simulink library "adeye_lib"  (R2019a)
settings: Solver=VariableStepAuto  StartTime=0.0  StopTime=10.0  RelTol=1e-3
undefined symbols (not defined in the file): AngularVelocity, Clock_, Data, Data_SL_Info, DiscIntNeverNeededParam, Encoding, Encoding_SL_Info, Header, Height, LinearAcceleration, Orientation, Pose, Step, Twist, Width
libraries: robotlib x47, $bdroot x46, simulink_extras x12, dspsrcs4 x6, dspindex x6, robotcorelib x2, aerolibutil x2, PreScanSimulinkLibrary x1
(part 2 of 4)

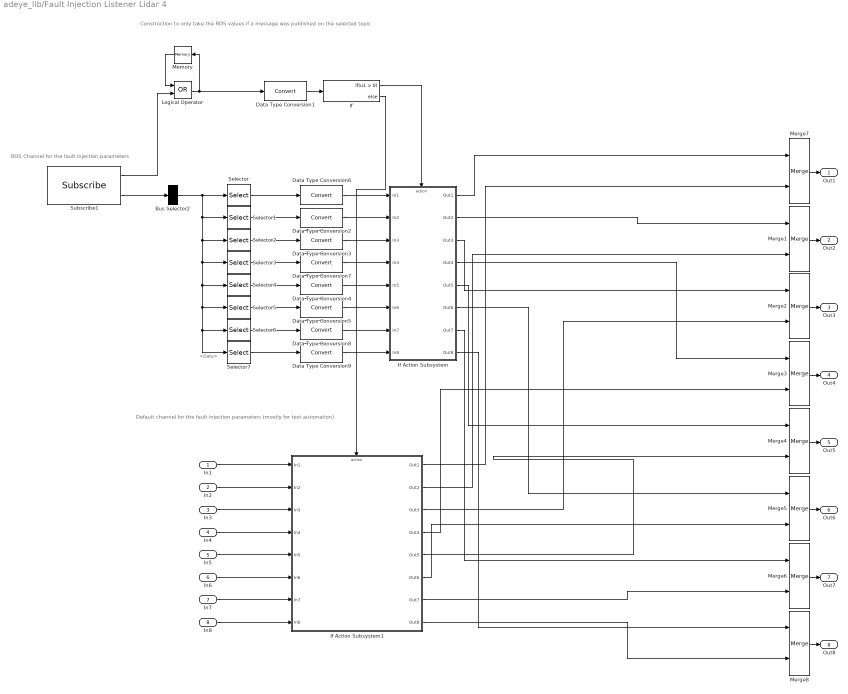
== system adeye_lib/Fault Injection Listener Lidar 4 ==
  note: Default channel for the fault injection parameters (mostly for test automation)
  note: ROS Channel for the fault injection parameters
  note: Construction to only take the ROS values if a message was published on the selected topic
  In1 : Inport
  In2 : Inport  Port=2
  In3 : Inport  Port=3
  In4 : Inport  Port=4
  In5 : Inport  Port=5
  In6 : Inport  Port=6
  In7 : Inport  Port=7
  In8 : Inport  Port=8
  Bus Selector2 : BusSelector  OutputSignals=Data
  Data Type Conversion{1..9} (9 alike) : DataTypeConversion
  If : If
  If Action Subsystem : Subsystem  TreatAsAtomicUnit=on
  If Action Subsystem1 : Subsystem  TreatAsAtomicUnit=on
  Logical Operator : Logic  Operator=OR  AllPortsSameDT=off  OutDataTypeStr=boolean
  Memory : Memory  InheritSampleTime=on
  Merge{1..8} (8 alike) : Merge
  Selector : Selector  InputPortWidth=128  IndexOptions=Index vector (dialog)  Indices=[1]  OutputSizes=1
  Selector1 : Selector  InputPortWidth=128  IndexOptions=Index vector (dialog)  Indices=[2]  OutputSizes=1
  Selector2 : Selector  InputPortWidth=128  IndexOptions=Index vector (dialog)  Indices=[3]  OutputSizes=1
  Selector3 : Selector  InputPortWidth=128  IndexOptions=Index vector (dialog)  Indices=[4]  OutputSizes=1
  Selector4 : Selector  InputPortWidth=128  IndexOptions=Index vector (dialog)  Indices=[5]  OutputSizes=1
  Selector5 : Selector  InputPortWidth=128  IndexOptions=Index vector (dialog)  Indices=[6]  OutputSizes=1
  Selector6 : Selector  InputPortWidth=128  IndexOptions=Index vector (dialog)  Indices=[7]  OutputSizes=1
  Selector7 : Selector  InputPortWidth=128  IndexOptions=Index vector (dialog)  Indices=[8]  OutputSizes=1
  Subscribe1 : robotlib/Subscribe  topicSource=Specify your own  topic=/fault_injection/lidar4  messageType=std_msgs/Float64MultiArray  sampleTime=-1  messageQueueLength=1
      settings: SourceProductBaseCode=RO
  Out1 : Outport
  Out2 : Outport  Port=2
  Out3 : Outport  Port=3
  Out4 : Outport  Port=4
  Out5 : Outport  Port=5
  Out6 : Outport  Port=6
  Out7 : Outport  Port=7
  Out8 : Outport  Port=8
  wires:
  Data Type Conversion6/1 -> If Action Subsystem/1(In1)
  If Action Subsystem/1(Out1) -> Merge7/1
  If/2 -> If Action Subsystem1/Action
  Logical Operator/1 -> Data Type Conversion1/1, Memory/1
  Subscribe1/1 -> Logical Operator/2
  Memory/1 -> Logical Operator/1
  If/1 -> If Action Subsystem/Action
  Data Type Conversion1/1 -> If/1
  If Action Subsystem1/1(Out1) -> Merge7/2
  Subscribe1/2 -> Bus Selector2/1
  In1/1 -> If Action Subsystem1/1(In1)
  Merge7/1 -> Out1/1
  Merge1/1 -> Out2/1
  Merge2/1 -> Out3/1
  Merge3/1 -> Out4/1
  Merge4/1 -> Out5/1
  Merge5/1 -> Out6/1
  Merge6/1 -> Out7/1
  Merge8/1 -> Out8/1
  If Action Subsystem/2(Out2) -> Merge1/1
  If Action Subsystem/3(Out3) -> Merge2/1
  If Action Subsystem/4(Out4) -> Merge3/1
  If Action Subsystem/5(Out5) -> Merge4/1
  If Action Subsystem/6(Out6) -> Merge5/1
  If Action Subsystem/7(Out7) -> Merge6/1
  If Action Subsystem/8(Out8) -> Merge8/1
  If Action Subsystem1/8(Out8) -> Merge8/2
  If Action Subsystem1/7(Out7) -> Merge6/2
  If Action Subsystem1/6(Out6) -> Merge5/2
  If Action Subsystem1/5(Out5) -> Merge4/2
  If Action Subsystem1/4(Out4) -> Merge3/2
  If Action Subsystem1/3(Out3) -> Merge2/2
  If Action Subsystem1/2(Out2) -> Merge1/2
  In2/1 -> If Action Subsystem1/2(In2)
  In5/1 -> If Action Subsystem1/5(In5)
  In4/1 -> If Action Subsystem1/4(In4)
  In3/1 -> If Action Subsystem1/3(In3)
  In6/1 -> If Action Subsystem1/6(In6)
  In8/1 -> If Action Subsystem1/8(In8)
  In7/1 -> If Action Subsystem1/7(In7)
  Data Type Conversion2/1 -> If Action Subsystem/2(In2)
  Selector1/1 -> Data Type Conversion2/1
  Data Type Conversion3/1 -> If Action Subsystem/3(In3)
  Selector2/1 -> Data Type Conversion3/1
  Data Type Conversion9/1 -> If Action Subsystem/8(In8)
  Data Type Conversion8/1 -> If Action Subsystem/7(In7)
  Data Type Conversion5/1 -> If Action Subsystem/6(In6)
  Data Type Conversion4/1 -> If Action Subsystem/5(In5)
  Data Type Conversion7/1 -> If Action Subsystem/4(In4)
  Selector3/1 -> Data Type Conversion7/1
  Selector4/1 -> Data Type Conversion4/1
  Selector5/1 -> Data Type Conversion5/1
  Selector6/1 -> Data Type Conversion8/1
  Selector7/1 -> Data Type Conversion9/1
  Selector/1 -> Data Type Conversion6/1
  Bus Selector2/1 -> Selector7/1, Selector6/1, Selector5/1, Selector4/1, Selector3/1, Selector2/1, Selector1/1, Selector/1  "<Data>"

== system adeye_lib/Fault Injection Listener Radar ==
  note: Default channel for the fault injection parameters (mostly for test automation)
  note: ROS Channel for the fault injection parameters
  note: Construction to only take the ROS values if a message was published on the selected topic
  State : Inport
  range_variance : Inport  Port=2
  theta_variance : Inport  Port=3
  phi_variance : Inport  Port=4
  Bus Selector2 : BusSelector  OutputSignals=Data
  Data Type Conversion{1..4,6} (5 alike) : DataTypeConversion
  If : If
  If Action Subsystem : Subsystem  TreatAsAtomicUnit=on
  If Action Subsystem1 : Subsystem  TreatAsAtomicUnit=on
  Logical Operator : Logic  Operator=OR  AllPortsSameDT=off  OutDataTypeStr=boolean
  Memory : Memory  InheritSampleTime=on
  Merge{1..3,7} (4 alike) : Merge
  Selector{,1..3} (4 alike) : Selector  InputPortWidth=128  IndexOptions=Index vector (dialog)  Indices=[1]  OutputSizes=1
  Subscribe1 : robotlib/Subscribe  topicSource=Specify your own  topic=/fault_injection/radar  messageType=std_msgs/Float64MultiArray  sampleTime=-1  messageQueueLength=1
      settings: SourceProductBaseCode=RO
  Out1 : Outport
  Out2 : Outport  Port=2
  Out3 : Outport  Port=3
  Out4 : Outport  Port=4
  wires:
  Merge7/1 -> Out1/1
  State/1 -> If Action Subsystem1/1(In1)
  Subscribe1/2 -> Bus Selector2/1
  If Action Subsystem1/1(Out1) -> Merge7/2
  Data Type Conversion1/1 -> If/1
  If/1 -> If Action Subsystem/Action
  Memory/1 -> Logical Operator/1
  Subscribe1/1 -> Logical Operator/2
  Logical Operator/1 -> Memory/1, Data Type Conversion1/1
  If/2 -> If Action Subsystem1/Action
  If Action Subsystem/1(Out1) -> Merge7/1
  Data Type Conversion6/1 -> If Action Subsystem/1(In1)
  Selector/1 -> Data Type Conversion6/1
  Bus Selector2/1 -> Selector3/1, Selector2/1, Selector1/1, Selector/1  "<Data>"
  Merge1/1 -> Out2/1
  Merge2/1 -> Out3/1
  Merge3/1 -> Out4/1
  If Action Subsystem/2(Out2) -> Merge1/1
  If Action Subsystem/3(Out3) -> Merge2/1
  If Action Subsystem/4(Out4) -> Merge3/1
  If Action Subsystem1/2(Out2) -> Merge1/2
  If Action Subsystem1/3(Out3) -> Merge2/2
  If Action Subsystem1/4(Out4) -> Merge3/2
  Selector1/1 -> Data Type Conversion2/1
  Selector2/1 -> Data Type Conversion3/1
  Data Type Conversion2/1 -> If Action Subsystem/2(In2)
  Data Type Conversion3/1 -> If Action Subsystem/3(In3)
  Selector3/1 -> Data Type Conversion4/1
  Data Type Conversion4/1 -> If Action Subsystem/4(In4)
  range_variance/1 -> If Action Subsystem1/2(In2)
  theta_variance/1 -> If Action Subsystem1/3(In3)
  phi_variance/1 -> If Action Subsystem1/4(In4)

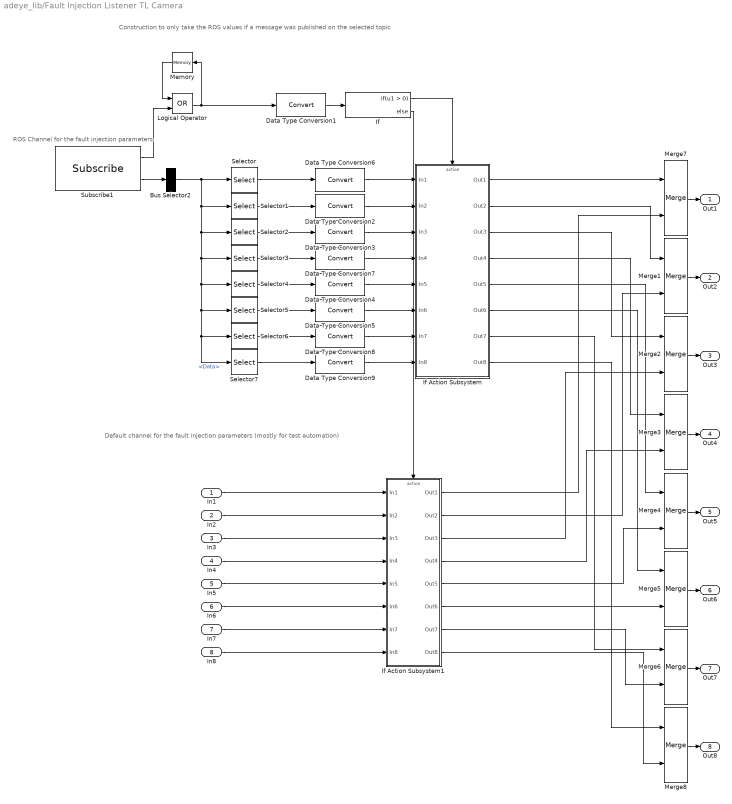
== system adeye_lib/Fault Injection Listener TL Camera ==
  note: Default channel for the fault injection parameters (mostly for test automation)
  note: ROS Channel for the fault injection parameters
  note: Construction to only take the ROS values if a message was published on the selected topic
  In1 : Inport
  In2 : Inport  Port=2
  In3 : Inport  Port=3
  In4 : Inport  Port=4
  In5 : Inport  Port=5
  In6 : Inport  Port=6
  In7 : Inport  Port=7
  In8 : Inport  Port=8
  Bus Selector2 : BusSelector  OutputSignals=Data
  Data Type Conversion{1..9} (9 alike) : DataTypeConversion
  If : If
  If Action Subsystem : Subsystem  TreatAsAtomicUnit=on
  If Action Subsystem1 : Subsystem  TreatAsAtomicUnit=on
  Logical Operator : Logic  Operator=OR  AllPortsSameDT=off  OutDataTypeStr=boolean
  Memory : Memory  InheritSampleTime=on
  Merge{1..8} (8 alike) : Merge
  Selector : Selector  InputPortWidth=128  IndexOptions=Index vector (dialog)  Indices=[1]  OutputSizes=1
  Selector1 : Selector  InputPortWidth=128  IndexOptions=Index vector (dialog)  Indices=[2]  OutputSizes=1
  Selector2 : Selector  InputPortWidth=128  IndexOptions=Index vector (dialog)  Indices=[3]  OutputSizes=1
  Selector3 : Selector  InputPortWidth=128  IndexOptions=Index vector (dialog)  Indices=[4]  OutputSizes=1
  Selector4 : Selector  InputPortWidth=128  IndexOptions=Index vector (dialog)  Indices=[5]  OutputSizes=1
  Selector5 : Selector  InputPortWidth=128  IndexOptions=Index vector (dialog)  Indices=[6]  OutputSizes=1
  Selector6 : Selector  InputPortWidth=128  IndexOptions=Index vector (dialog)  Indices=[7]  OutputSizes=1
  Selector7 : Selector  InputPortWidth=128  IndexOptions=Index vector (dialog)  Indices=[8]  OutputSizes=1
  Subscribe1 : robotlib/Subscribe  topicSource=Specify your own  topic=/fault_injection/tl_camera  messageType=std_msgs/Float64MultiArray  sampleTime=-1  messageQueueLength=1
      settings: SourceProductBaseCode=RO
  Out1 : Outport
  Out2 : Outport  Port=2
  Out3 : Outport  Port=3
  Out4 : Outport  Port=4
  Out5 : Outport  Port=5
  Out6 : Outport  Port=6
  Out7 : Outport  Port=7
  Out8 : Outport  Port=8
  wires:
  If Action Subsystem/1(Out1) -> Merge7/1
  If/2 -> If Action Subsystem1/Action
  Logical Operator/1 -> Data Type Conversion1/1, Memory/1
  Subscribe1/1 -> Logical Operator/2
  Memory/1 -> Logical Operator/1
  If/1 -> If Action Subsystem/Action
  Data Type Conversion1/1 -> If/1
  If Action Subsystem1/1(Out1) -> Merge7/2
  Subscribe1/2 -> Bus Selector2/1
  In1/1 -> If Action Subsystem1/1(In1)
  Merge7/1 -> Out1/1
  Selector/1 -> Data Type Conversion6/1
  Selector7/1 -> Data Type Conversion9/1
  Selector6/1 -> Data Type Conversion8/1
  Data Type Conversion4/1 -> If Action Subsystem/5(In5)
  Selector5/1 -> Data Type Conversion5/1
  Selector3/1 -> Data Type Conversion7/1
  Data Type Conversion5/1 -> If Action Subsystem/6(In6)
  Data Type Conversion7/1 -> If Action Subsystem/4(In4)
  Data Type Conversion8/1 -> If Action Subsystem/7(In7)
  Bus Selector2/1 -> Selector7/1, Selector6/1, Selector5/1, Selector4/1, Selector3/1, Selector2/1, Selector1/1, Selector/1  "<Data>"
  Data Type Conversion9/1 -> If Action Subsystem/8(In8)
  Selector4/1 -> Data Type Conversion4/1
  Selector1/1 -> Data Type Conversion2/1
  Data Type Conversion2/1 -> If Action Subsystem/2(In2)
  Data Type Conversion6/1 -> If Action Subsystem/1(In1)
  Selector2/1 -> Data Type Conversion3/1
  Data Type Conversion3/1 -> If Action Subsystem/3(In3)
  In2/1 -> If Action Subsystem1/2(In2)
  In3/1 -> If Action Subsystem1/3(In3)
  In4/1 -> If Action Subsystem1/4(In4)
  In5/1 -> If Action Subsystem1/5(In5)
  In6/1 -> If Action Subsystem1/6(In6)
  In7/1 -> If Action Subsystem1/7(In7)
  In8/1 -> If Action Subsystem1/8(In8)
  Merge1/1 -> Out2/1
  Merge2/1 -> Out3/1
  Merge3/1 -> Out4/1
  Merge4/1 -> Out5/1
  Merge5/1 -> Out6/1
  Merge6/1 -> Out7/1
  Merge8/1 -> Out8/1
  If Action Subsystem1/8(Out8) -> Merge8/2
  If Action Subsystem1/7(Out7) -> Merge6/2
  If Action Subsystem1/6(Out6) -> Merge5/2
  If Action Subsystem1/5(Out5) -> Merge4/2
  If Action Subsystem1/4(Out4) -> Merge3/2
  If Action Subsystem1/3(Out3) -> Merge2/2
  If Action Subsystem1/2(Out2) -> Merge1/2
  If Action Subsystem/2(Out2) -> Merge1/1
  If Action Subsystem/3(Out3) -> Merge2/1
  If Action Subsystem/8(Out8) -> Merge8/1
  If Action Subsystem/4(Out4) -> Merge3/1
  If Action Subsystem/5(Out5) -> Merge4/1
  If Action Subsystem/6(Out6) -> Merge5/1
  If Action Subsystem/7(Out7) -> Merge6/1

== system adeye_lib/Fault Injection Radar ==
  Range : Inport
  Theta : Inport  Port=2
  Phi : Inport  Port=3
  TargetTypeID : Inport  Port=4
  On/Off : Inport  Port=5
  range_variance : Inport  Port=6
  theta_variance : Inport  Port=7
  phi_variance : Inport  Port=8
  If : If
  If Action Subsystem : Subsystem  TreatAsAtomicUnit=on
  If Action Subsystem1 : Subsystem  TreatAsAtomicUnit=on
  Merge{,1..3} (4 alike) : Merge
  Out1 : Outport
  Out2 : Outport  Port=2
  Out3 : Outport  Port=3
  Out4 : Outport  Port=4
  wires:
  Merge/1 -> Out1/1
  Merge1/1 -> Out2/1
  Merge2/1 -> Out3/1
  If Action Subsystem/4(Out4) -> Merge3/1
  If Action Subsystem/3(Out3) -> Merge2/1
  If Action Subsystem/2(Out2) -> Merge1/1
  If Action Subsystem/1(Out1) -> Merge/1
  If Action Subsystem1/1(Out1) -> Merge/2
  If Action Subsystem1/2(Out2) -> Merge1/2
  If Action Subsystem1/3(Out3) -> Merge2/2
  If Action Subsystem1/4(Out4) -> Merge3/2
  Merge3/1 -> Out4/1
  On/Off/1 -> If/1
  TargetTypeID/1 -> If Action Subsystem1/4(In4), If Action Subsystem/4(In4)
  Phi/1 -> If Action Subsystem1/3(phi), If Action Subsystem/3(In3)
  Theta/1 -> If Action Subsystem/2(In2), If Action Subsystem1/2(theta)
  Range/1 -> If Action Subsystem1/1(range), If Action Subsystem/1(In1)
  If/1 -> If Action Subsystem1/Action
  If/2 -> If Action Subsystem/Action
  range_variance/1 -> If Action Subsystem1/5(range_variance)
  theta_variance/1 -> If Action Subsystem1/6(theta_variance)
  phi_variance/1 -> If Action Subsystem1/7(phi_variance)

== system adeye_lib/Lidar Adapter ==
  In1 : Inport
  In2 : Inport  Port=2
  In3 : Inport  Port=3
  In4 : Inport  Port=4
  In5 : Inport  Port=5
  Matrix Concatenate5 : Concatenate  NumInputs=4  Mode=Multidimensional array  ConcatenateDimension=2
  Reshape{1..4} (4 alike) : Reshape
  Rotate over Z : Subsystem
  Spherical to cartesian : Subsystem
  Out1 : Outport
  wires:
  In4/1 -> Reshape2/1
  In2/1 -> Reshape4/1
  Matrix Concatenate5/1 -> Out1/1
  Rotate over Z/1(Out1) -> Matrix Concatenate5/1
  Reshape3/1 -> Matrix Concatenate5/4
  Spherical to cartesian/3(Out3) -> Matrix Concatenate5/3
  Rotate over Z/2(Out2) -> Matrix Concatenate5/2
  In3/1 -> Reshape1/1
  Spherical to cartesian/2(Out2) -> Rotate over Z/3(In3)
  Reshape2/1 -> Spherical to cartesian/3(In3)
  Spherical to cartesian/1(Out1) -> Rotate over Z/2(In2)
  Reshape1/1 -> Spherical to cartesian/2(In2)
  In1/1 -> Rotate over Z/1(In1)
  Reshape4/1 -> Spherical to cartesian/1(In1)
  In5/1 -> Reshape3/1

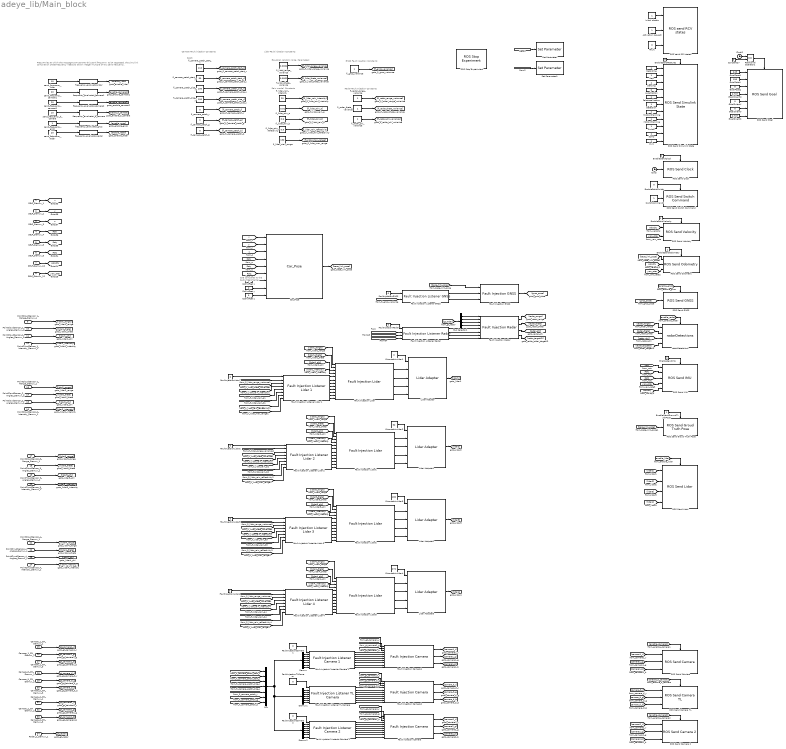
== system adeye_lib/Main_block ==
  note: Rain model, Constants
  note: Patch
  note: Lidar Fault injection Constants
  note: Camera Fault injection Constants
  note: Radar Fault Injection Constants
  note: Gaussian random noise, Parameters
  note: GNSS Fault Injection Constants
  note: CoG  compared
      | to the backwheels
      | center
  note: Frequencies at which the messages are sent
      |
      | For this send frequency to be respected, the simulink compilation sheet frequency
      | needs to be an integer multiple of this send frequency.
  SELF_Demux_1 : Inport
  SELF_Demux_2 : Inport  Port=2
  SELF_Demux_3 : Inport  Port=3
  SELF_Demux_4 : Inport  Port=4
  SELF_Demux_5 : Inport  Port=5
  SELF_Demux_6 : Inport  Port=6
  SELF_Demux_10 : Inport  Port=7
  SELF_Demux_12 : Inport  Port=8
  PointCloudSensor_1_Range_Demux_1 : Inport  Port=9
  PointCloudSensor_1_Angles_Demux_1 : Inport  Port=10
  PointCloudSensor_1_Angles_Demux_2 : Inport  Port=11
  PointCloudSensor_1_Intensity_Demux_1 : Inport  Port=12
  PointCloudSensor_2_Range_Demux_1 : Inport  Port=13
  PointCloudSensor_2_Angles_Demux_1 : Inport  Port=14
  PointCloudSensor_2_Angles_Demux_2 : Inport  Port=15
  PointCloudSensor_2_Intensity_Demux_1 : Inport  Port=16
  PointCloudSensor_3_Range_Demux_1 : Inport  Port=17
  PointCloudSensor_3_Angles_Demux_1 : Inport  Port=18
  PointCloudSensor_3_Angles_Demux_2 : Inport  Port=19
  PointCloudSensor_3_Intensity_Demux_1 : Inport  Port=20
  PointCloudSensor_4_Range_Demux_1 : Inport  Port=21
  PointCloudSensor_4_Angles_Demux_1 : Inport  Port=22
  PointCloudSensor_4_Angles_Demux_2 : Inport  Port=23
  PointCloudSensor_4_Intensity_Demux_1 : Inport  Port=24
  Camera_1_CM_Demux_1 : Inport  Port=25
  Camera_1_CM_Demux_2 : Inport  Port=26
  Camera_1_CM_Demux_3 : Inport  Port=27
  Camera_tl_CM_Demux_1 : Inport  Port=28
  Camera_tl_CM_Demux_2 : Inport  Port=29
  Camera_tl_CM_Demux_3 : Inport  Port=30
  Camera_2_CM_Demux_1 : Inport  Port=31
  Camera_2_CM_Demux_2 : Inport  Port=32
  Camera_2_CM_Demux_3 : Inport  Port=33
  Radar_1_Demux_1 : Inport  Port=34
  Activation request : Constant  OutDataTypeStr=Inherit: Inherit via back propagation
  Bus Selector1 : BusSelector  OutputSignals=Range[m],Theta[deg],Phi[deg],TargetTypeID[-]
  Car_Pose : $bdroot/Car_Pose  SystemSampleTime=-1
  Clock : Clock
  Clock2 : Clock
  CoG offset x : Constant  Value=0
  CoG offset y : Constant  Value=0
  CoG offset z : Constant  Value=0
  Constant27 : Constant  Value=0
  Demux : Demux  Outputs=7
  Demux1 : Demux  Outputs=7
  Demux2 : Demux  Outputs=7
  Detection : Constant
  EnableSendClock : Constant  OutDataTypeStr=Inherit: Inherit via back propagation
  EnableSendFeatures : Constant  Value=0  OutDataTypeStr=Inherit: Inherit via back propagation
  EnableSendGroundTruthPose : Constant
  EnableSendIMU : Constant  OutDataTypeStr=Inherit: Inherit via back propagation
  EnableSendOdometry : Constant
  EnableSendSwitch : Constant  Value=0  OutDataTypeStr=Inherit: Inherit via back propagation  SampleTime=0.05
  EnableSendVelocity : Constant  OutDataTypeStr=Inherit: Inherit via back propagation
  FakeLocalization : Constant
  Fault : Constant  Value=0  OutDataTypeStr=Inherit: Inherit via back propagation
  Fault Injection Camera : $bdroot/Fault Injection Camera  idy=200  idx=100  x=100  y=150  R=0  G=0  B=0
  Fault Injection Camera1 : $bdroot/Fault Injection Camera  idy=200  idx=100  x=100  y=150  R=0  G=0  B=0
  Fault Injection Camera2 : $bdroot/Fault Injection Camera  idy=200  idx=100  x=100  y=150  R=0  G=0  B=0
  Fault Injection GNSS : $bdroot/Fault Injection GNSS  f=20
  Fault Injection Lidar{,1..3} (4 alike) : $bdroot/Fault Injection Lidar  f=20  p=225*16
  Fault Injection Listener Camera 1 : $bdroot/Fault Injection Listener Camera 1  SystemSampleTime=-1
  Fault Injection Listener Camera 2 : $bdroot/Fault Injection Listener Camera 2  SystemSampleTime=-1
  Fault Injection Listener GNSS : $bdroot/Fault Injection Listener GNSS  SystemSampleTime=-1
  Fault Injection Listener Lidar 1 : $bdroot/Fault Injection Listener Lidar 1  SystemSampleTime=-1
  Fault Injection Listener Lidar 2 : $bdroot/Fault Injection Listener Lidar 2  SystemSampleTime=-1
  Fault Injection Listener Lidar 3 : $bdroot/Fault Injection Listener Lidar 3  SystemSampleTime=-1
  Fault Injection Listener Lidar 4 : $bdroot/Fault Injection Listener Lidar 4  SystemSampleTime=-1
  Fault Injection Listener Radar : $bdroot/Fault Injection Listener Radar  SystemSampleTime=-1
  Fault Injection Listener TL Camera : $bdroot/Fault Injection Listener TL Camera  SystemSampleTime=-1
  Fault Injection Radar : $bdroot/Fault Injection Radar  n=7
  FaultInjectionCamera1 : Constant  Value=0
  FaultInjectionCamera2 : Constant  Value=0
  FaultInjectionGNSS : Constant  Value=0  OutDataTypeStr=Inherit: Inherit via back propagation  SampleTime=0.05
  FaultInjectionLidar{1..4} (4 alike) : Constant  Value=0  OutDataTypeStr=Inherit: Inherit via back propagation
  FaultInjectionRadar : Constant  Value=0
  FaultInjectionTLCamera : Constant  Value=0
  GoalOrientW : Constant  Value=0.707
  GoalOrientX : Constant  Value=0
  GoalOrientY : Constant  Value=0
  GoalOrientZ : Constant  Value=0.707
  GoalPoseX : Constant  Value=249
  GoalPoseY : Constant  Value=136
  GoalPoseZ : Constant  Value=0
  Initial checks : Constant  OutDataTypeStr=Inherit: Inherit via back propagation
  Lidar Adapter{,1..3} (4 alike) : $bdroot/Lidar Adapter  SystemSampleTime=-1
  Localization : Constant  Value=0
  Map : Constant
  MissionPlanning : Constant
  MotionPlanning : Constant
  Mux : Mux  Inputs=7
  OrientationLidar1 : Constant  Value=0  OutDataTypeStr=Inherit: Inherit via back propagation
  OrientationLidar2 : Constant  Value=90  OutDataTypeStr=Inherit: Inherit via back propagation
  OrientationLidar3 : Constant  Value=180  OutDataTypeStr=Inherit: Inherit via back propagation
  OrientationLidar4 : Constant  Value=270  OutDataTypeStr=Inherit: Inherit via back propagation
  ROS Send Camera : $bdroot/ROS Send Camera  SystemSampleTime=-1
  ROS Send Camera 2 : $bdroot/ROS Send Camera 2  SystemSampleTime=-1
  ROS Send Camera TL : $bdroot/ROS Send Camera TL  SystemSampleTime=-1
  ROS Send Clock : $bdroot/ROS Send Clock  Priority=1  SystemSampleTime=-1
  ROS Send GNSS : $bdroot/ROS Send GNSS  SystemSampleTime=-1
  ROS Send Goal : $bdroot/ROS Send Goal  SystemSampleTime=-1
  ROS Send Groud Truth Pose : $bdroot/ROS Send Groud Truth Pose  SystemSampleTime=-1
  ROS Send IMU : $bdroot/ROS Send IMU  SystemSampleTime=-1
  ROS Send Lidar : $bdroot/ROS Send Lidar  SystemSampleTime=-1
  ROS Send Odometry : $bdroot/ROS Send Odometry  SystemSampleTime=-1
  ROS Send Simulink State : $bdroot/ROS Send Simulink State  SystemSampleTime=-1
  ROS Send Switch Command : $bdroot/ROS Send Switch Command  SystemSampleTime=-1
  ROS Send Velocity : $bdroot/ROS Send Velocity  SystemSampleTime=-1
  ROS Stop Experiment : $bdroot/ROS Stop Experiment  SystemSampleTime=-1
  ROS send RCV states : $bdroot/ROS send RCV states  SystemSampleTime=-1
  Recording : Constant
  Relational Operator1 : RelationalOperator  Operator===  OutDataTypeStr=boolean  RndMeth=Simplest
  Rviz : Constant
  Sensing : Constant
  Set Parameter : robotlib/Set Parameter  ParameterSource=Specify your own  ParameterName=/simulink/rain_intensity  ParameterType=double  ModelName=ROS_lib  BlockId=ParamSet_ROS_lib_3479
      settings: SourceProductName=Robotics System Toolbox  SourceProductBaseCode=RO
  Set Parameter1 : robotlib/Set Parameter  ParameterSource=Specify your own  ParameterName=/simulink/reflectivity  ParameterType=double  ModelName=ROS_lib  BlockId=ParamSet_ROS_lib_3480
      settings: SourceProductName=Robotics System Toolbox  SourceProductBaseCode=RO
  Ssmp : Constant
  Switch : Constant
  SwitchCommand : Constant  OutDataTypeStr=Inherit: Inherit via back propagation  SampleTime=0.05
  fi_camera_patch_b : Constant  Value=0
  fi_camera_patch_g : Constant  Value=0
  fi_camera_patch_r : Constant  Value=0
  fi_camera_patch_size_x : Constant  Value=100
  fi_camera_patch_size_y : Constant  Value=100
  fi_camera_patch_start_x : Constant  Value=110
  fi_camera_patch_start_y : Constant  Value=50
  fi_gnss_variance : Constant
  fi_lidar_max_range : Constant  Value=150
  fi_lidar_rain_a : Constant  Value=0.01
  fi_lidar_rain_b : Constant  Value=0.6
  fi_lidar_rain_intensity : Constant  Value=20
  fi_lidar_rain_reflectivity : Constant  Value=0.9
  fi_lidar_range_variance : Constant  Value=0.0001
  fi_lidar_theta_variance : Constant  Value=0.0001
  fi_radar_phi_variance : Constant
  fi_radar_range_variance : Constant
  fi_radar_theta_variance : Constant
  frequency_evaluator_camera1 : $bdroot/frequency_evaluator  SystemSampleTime=-1
  frequency_evaluator_camera2 : $bdroot/frequency_evaluator  SystemSampleTime=-1
  frequency_evaluator_gnss : $bdroot/frequency_evaluator  SystemSampleTime=-1
  frequency_evaluator_lidar : $bdroot/frequency_evaluator  SystemSampleTime=-1
      link override Constant: Value=0.999
  frequency_evaluator_radar : $bdroot/frequency_evaluator  SystemSampleTime=-1
  frequency_evaluator_tl_camera : $bdroot/frequency_evaluator  SystemSampleTime=-1
  radarDetections : $bdroot/radarDetections  SystemSampleTime=-1
  send_frequency_camera1 : Constant  Priority=1  Value=20
  send_frequency_camera2 : Constant  Priority=1  Value=20
  send_frequency_gnss : Constant  Priority=1
  send_frequency_lidar : Constant  Priority=1  Value=10
  send_frequency_radar : Constant  Priority=1  Value=20
  send_frequency_tl_camera : Constant  Priority=1  Value=10
  tag scope: Rotx=global, Roty=global, Rotz=global, velocity=global, x=global, y=global, yaw_rate=global, z=global
  wires:
  [p_refl_sfc] -> Set Parameter1/1
  [rain_intensity] -> Set Parameter/1
  Radar_1_Demux_1/1 -> [gt_radar]
  Camera_2_CM_Demux_3/1 -> [gt_camera2_b]
  Camera_2_CM_Demux_2/1 -> [gt_camera2_g]
  Camera_2_CM_Demux_1/1 -> [gt_camera2_r]
  SELF_Demux_10/1 -> [velocity]
  SELF_Demux_5/1 -> [Roty]
  SELF_Demux_12/1 -> [yaw_rate]
  SELF_Demux_4/1 -> [Rotx]
  SELF_Demux_1/1 -> [x]
  SELF_Demux_6/1 -> [Rotz]
  SELF_Demux_2/1 -> [y]
  SELF_Demux_3/1 -> [z]
  Camera_1_CM_Demux_1/1 -> [gt_camera1_r]
  Camera_1_CM_Demux_2/1 -> [gt_camera1_g]
  Camera_tl_CM_Demux_3/1 -> [gt_camera_tl_b]
  Camera_tl_CM_Demux_2/1 -> [gt_camera_tl_g]
  Camera_1_CM_Demux_3/1 -> [gt_camera1_b]
  Camera_tl_CM_Demux_1/1 -> [gt_camera_tl_r]
  GoalOrientW/1 -> ROS Send Goal/4
  GoalOrientX/1 -> ROS Send Goal/5
  GoalOrientY/1 -> ROS Send Goal/6
  Constant27/1 -> Relational Operator1/2
  Relational Operator1/1 -> ROS Send Goal/Enable
  Clock2/1 -> Relational Operator1/1
  GoalPoseZ/1 -> ROS Send Goal/3
  GoalPoseY/1 -> ROS Send Goal/2
  GoalOrientZ/1 -> ROS Send Goal/7
  GoalPoseX/1 -> ROS Send Goal/1
  EnableSendFeatures/1 -> ROS Send Simulink State/Enable
  [camera1_g] -> ROS Send Camera/2
  [camera1_b] -> ROS Send Camera/3
  [radar_phi] -> radarDetections/3
  [radar_range] -> radarDetections/1
  [velocity] -> ROS Send Odometry/2
  [gnss_pose] -> ROS Send GNSS/1
  MissionPlanning/1 -> ROS Send Simulink State/7
  [velocity] -> ROS Send Velocity/1
  EnableSendClock/1 -> ROS Send Clock/Enable
  Localization/1 -> ROS Send Simulink State/4
  Detection/1 -> ROS Send Simulink State/6
  FakeLocalization/1 -> ROS Send Simulink State/5
  [camera2_b] -> ROS Send Camera 2/3
  MotionPlanning/1 -> ROS Send Simulink State/8
  [camera1_r] -> ROS Send Camera/1
  [velocity] -> ROS Send IMU/5
  [camera_tl_b] -> ROS Send Camera TL/3
  [camera2_g] -> ROS Send Camera 2/2
  [camera2_r] -> ROS Send Camera 2/1
  [camera_tl_r] -> ROS Send Camera TL/1
  SwitchCommand/1 -> ROS Send Switch Command/1
  EnableSendVelocity/1 -> ROS Send Velocity/Enable
  Rviz/1 -> ROS Send Simulink State/11
  Switch/1 -> ROS Send Simulink State/9
  Recording/1 -> ROS Send Simulink State/1
  EnableSendOdometry/1 -> ROS Send Odometry/Enable
  Activation request/1 -> ROS send RCV states/2
  EnableSendSwitch/1 -> ROS Send Switch Command/Enable
  EnableSendIMU/1 -> ROS Send IMU/Enable
  [radar_targetID] -> radarDetections/4
  [yaw_rate] -> ROS Send IMU/4
  [lidar4] -> ROS Send Lidar/4
  Sensing/1 -> ROS Send Simulink State/3
  [yaw_rate] -> ROS Send Velocity/2
  [camera_tl_g] -> ROS Send Camera TL/2
  [Rotz] -> ROS Send IMU/3
  Fault/1 -> ROS send RCV states/3
  [Roty] -> ROS Send IMU/2
  Ssmp/1 -> ROS Send Simulink State/10
  [Rotx] -> ROS Send IMU/1
  [lidar2] -> ROS Send Lidar/2
  [radar_theta] -> radarDetections/2
  [yaw_rate] -> ROS Send Odometry/3
  [lidar3] -> ROS Send Lidar/3
  Clock/1 -> ROS Send Clock/1
  Map/1 -> ROS Send Simulink State/2
  Initial checks/1 -> ROS send RCV states/1
  [lidar1] -> ROS Send Lidar/1
  [base_link_pose] -> ROS Send Odometry/1
  fi_camera_patch_start_x/1 -> [fi_camera_patch_start_x]
  fi_camera_patch_start_y/1 -> [fi_camera_patch_start_y]
  fi_camera_patch_size_x/1 -> [fi_camera_patch_size_x]
  fi_radar_range_variance/1 -> [fi_radar_range_variance]
  fi_radar_theta_variance/1 -> [fi_radar_theta_variance]
  fi_lidar_range_variance/1 -> [fi_lidar_range_variance]
  fi_lidar_theta_variance/1 -> [fi_lidar_theta_variance]
  fi_radar_phi_variance/1 -> [fi_radar_phi_variance]
  fi_gnss_variance/1 -> [fi_gnss_variance]
  fi_camera_patch_g/1 -> [fi_camera_patch_g]
  fi_camera_patch_b/1 -> [fi_camera_patch_b]
  fi_lidar_rain_reflectivity/1 -> [fi_lidar_rain_reflectivity]
  fi_lidar_max_range/1 -> [fi_lidar_max_range]
  fi_camera_patch_r/1 -> [fi_camera_patch_r]
  fi_lidar_rain_a/1 -> [fi_lidar_rain_a]
  fi_lidar_rain_intensity/1 -> [fi_lidar_rain_intensity]
  fi_camera_patch_size_y/1 -> [fi_camera_patch_size_y]
  fi_lidar_rain_b/1 -> [fi_lidar_rain_b]
  PointCloudSensor_1_Range_Demux_1/1 -> [lidar1_range]
  PointCloudSensor_1_Angles_Demux_1/1 -> [lidar1_theta]
  PointCloudSensor_1_Angles_Demux_2/1 -> [lidar1_phi]
  PointCloudSensor_1_Intensity_Demux_1/1 -> [lidar1_intensity]
  PointCloudSensor_2_Range_Demux_1/1 -> [lidar2_range]
  PointCloudSensor_2_Angles_Demux_1/1 -> [lidar2_theta]
  PointCloudSensor_3_Range_Demux_1/1 -> [lidar3_range]
  PointCloudSensor_3_Angles_Demux_1/1 -> [lidar3_theta]
  PointCloudSensor_3_Angles_Demux_2/1 -> [lidar3_phi]
  PointCloudSensor_3_Intensity_Demux_1/1 -> [lidar3_intensity]
  PointCloudSensor_4_Range_Demux_1/1 -> [lidar4_range]
  PointCloudSensor_4_Angles_Demux_1/1 -> [lidar4_theta]
  PointCloudSensor_4_Intensity_Demux_1/1 -> [lidar4_intensity]
  PointCloudSensor_4_Angles_Demux_2/1 -> [lidar4_phi]
  PointCloudSensor_2_Angles_Demux_2/1 -> [lidar2_phi]
  PointCloudSensor_2_Intensity_Demux_1/1 -> [lidar2_intensity]
  OrientationLidar2/1 -> Lidar Adapter1/1
  Fault Injection Listener Radar/3 -> Fault Injection Radar/7
  Fault Injection Lidar3/4 -> Lidar Adapter3/5
  [fi_lidar_range_variance] -> Fault Injection Listener Lidar 3/2
  FaultInjectionLidar4/1 -> Fault Injection Listener Lidar 4/1
  [fi_lidar_rain_a] -> Fault Injection Listener Lidar 3/5
  [fi_lidar_theta_variance] -> Fault Injection Listener Lidar 4/3
  Fault Injection Camera/2 -> [camera2_g]
  Fault Injection Listener Lidar 4/2 -> Fault Injection Lidar3/6
  Fault Injection Camera2/3 -> [camera_tl_b]
  Fault Injection Camera1/1 -> [camera1_r]
  Fault Injection Camera/3 -> [camera2_b]
  [fi_lidar_rain_intensity] -> Fault Injection Listener Lidar 4/4
  [fi_lidar_rain_b] -> Fault Injection Listener Lidar 2/6
  Bus Selector1/4 -> Fault Injection Radar/4  "<TargetTypeID[-]>"
  [fi_lidar_rain_a] -> Fault Injection Listener Lidar 2/5
  Fault Injection Camera2/1 -> [camera_tl_r]
  [fi_lidar_rain_intensity] -> Fault Injection Listener Lidar 1/4
  Fault Injection Camera1/3 -> [camera1_b]
  Fault Injection Listener Lidar 3/6 -> Fault Injection Lidar2/10
  [lidar1_theta] -> Fault Injection Lidar/2
  [fi_lidar_max_range] -> Fault Injection Listener Lidar 1/8
  Fault Injection Camera2/2 -> [camera_tl_g]
  [lidar4_theta] -> Fault Injection Lidar3/2
  Fault Injection Listener Camera 2/3 -> Fault Injection Camera/6
  Fault Injection Lidar2/2 -> Lidar Adapter2/3
  Fault Injection Listener TL Camera/5 -> Fault Injection Camera2/8
  Fault Injection Radar/4 -> [radar_targetID]
  Fault Injection Radar/2 -> [radar_theta]
  [lidar1_phi] -> Fault Injection Lidar/3
  Fault Injection Listener Lidar 4/5 -> Fault Injection Lidar3/9
  [Roty] -> Car_Pose/5
  Fault Injection Listener Lidar 1/3 -> Fault Injection Lidar/7
  Fault Injection Listener Lidar 2/3 -> Fault Injection Lidar1/7
  [lidar2_theta] -> Fault Injection Lidar1/2
  [lidar4_phi] -> Fault Injection Lidar3/3
  Fault Injection Listener TL Camera/3 -> Fault Injection Camera2/6
  Fault Injection Listener Lidar 3/2 -> Fault Injection Lidar2/6
  Fault Injection Listener Camera 1/8 -> Fault Injection Camera1/11
  [lidar3_theta] -> Fault Injection Lidar2/2
  [lidar3_intensity] -> Fault Injection Lidar2/4
  Fault Injection Listener Lidar 3/1 -> Fault Injection Lidar2/5
  Bus Selector1/2 -> Fault Injection Radar/2  "<Theta[deg]>"
  Fault Injection Listener Lidar 2/7 -> Fault Injection Lidar1/11
  [gt_camera_tl_g] -> Fault Injection Camera2/2
  [lidar1_range] -> Fault Injection Lidar/1
  Fault Injection Lidar1/3 -> Lidar Adapter1/4
  [fi_lidar_rain_reflectivity] -> Fault Injection Listener Lidar 3/7
  [gt_camera_tl_r] -> Fault Injection Camera2/1
  [lidar3_range] -> Fault Injection Lidar2/1
  Fault Injection Listener Camera 1/6 -> Fault Injection Camera1/9
  Fault Injection Lidar2/3 -> Lidar Adapter2/4
  Lidar Adapter3/1 -> [lidar4]
  Fault Injection Listener Lidar 4/4 -> Fault Injection Lidar3/8
  [gt_camera_tl_b] -> Fault Injection Camera2/3
  Fault Injection Listener GNSS/2 -> Fault Injection GNSS/3
  Fault Injection Listener Lidar 2/8 -> Fault Injection Lidar1/12
  Fault Injection Lidar/3 -> Lidar Adapter/4
  Fault Injection Listener Radar/4 -> Fault Injection Radar/8
  [fi_radar_theta_variance] -> Fault Injection Listener Radar/3
  OrientationLidar4/1 -> Lidar Adapter3/1
  [fi_lidar_theta_variance] -> Fault Injection Listener Lidar 1/3
  Fault Injection Listener Camera 1/3 -> Fault Injection Camera1/6
  Fault Injection Listener Camera 1/4 -> Fault Injection Camera1/7
  Fault Injection Listener TL Camera/4 -> Fault Injection Camera2/7
  Fault Injection Radar/3 -> [radar_phi]
  Fault Injection Listener TL Camera/6 -> Fault Injection Camera2/9
  Fault Injection Listener Camera 2/2 -> Fault Injection Camera/5
  Fault Injection Listener Camera 2/4 -> Fault Injection Camera/7
  Fault Injection Listener Camera 2/5 -> Fault Injection Camera/8
  Fault Injection Listener Lidar 3/5 -> Fault Injection Lidar2/9
  Fault Injection Listener Lidar 1/5 -> Fault Injection Lidar/9
  Fault Injection Lidar3/3 -> Lidar Adapter3/4
  Fault Injection Listener Lidar 1/7 -> Fault Injection Lidar/11
  Fault Injection Listener Lidar 4/6 -> Fault Injection Lidar3/10
  Fault Injection Listener Lidar 4/1 -> Fault Injection Lidar3/5
  Fault Injection Listener Lidar 3/3 -> Fault Injection Lidar2/7
  Fault Injection Listener Camera 1/2 -> Fault Injection Camera1/5
  Fault Injection Lidar3/2 -> Lidar Adapter3/3
  Fault Injection Listener Camera 2/7 -> Fault Injection Camera/10
  Fault Injection Lidar3/1 -> Lidar Adapter3/2
  CoG offset z/1 -> Car_Pose/9
  Fault Injection Listener Lidar 2/4 -> Fault Injection Lidar1/8
  Fault Injection Listener Lidar 2/6 -> Fault Injection Lidar1/10
  Fault Injection Listener Lidar 2/5 -> Fault Injection Lidar1/9
  Fault Injection Lidar1/4 -> Lidar Adapter1/5
  Fault Injection Lidar2/4 -> Lidar Adapter2/5
  [fi_gnss_variance] -> Fault Injection Listener GNSS/2
  Fault Injection Lidar2/1 -> Lidar Adapter2/2
  Fault Injection Listener Lidar 1/6 -> Fault Injection Lidar/10
  Fault Injection Lidar1/1 -> Lidar Adapter1/2
  Fault Injection Listener Lidar 1/8 -> Fault Injection Lidar/12
  Fault Injection Listener Lidar 3/7 -> Fault Injection Lidar2/11
  Fault Injection Listener Lidar 1/4 -> Fault Injection Lidar/8
  Fault Injection Listener Lidar 2/1 -> Fault Injection Lidar1/5
  Fault Injection Lidar1/2 -> Lidar Adapter1/3
  [gt_camera2_g] -> Fault Injection Camera/2
  [lidar2_phi] -> Fault Injection Lidar1/3
  FaultInjectionRadar/1 -> Fault Injection Listener Radar/1
  Fault Injection Listener Lidar 3/4 -> Fault Injection Lidar2/8
  FaultInjectionCamera2/1 -> Fault Injection Listener Camera 2/1
  [gt_camera1_b] -> Fault Injection Camera1/3
  [gt_camera1_r] -> Fault Injection Camera1/1
  Fault Injection Listener Lidar 4/7 -> Fault Injection Lidar3/11
  Fault Injection Listener Lidar 1/2 -> Fault Injection Lidar/6
  [lidar2_range] -> Fault Injection Lidar1/1
  Fault Injection Listener Camera 2/1 -> Fault Injection Camera/4
  FaultInjectionCamera1/1 -> Fault Injection Listener Camera 1/1
  FaultInjectionTLCamera/1 -> Fault Injection Listener TL Camera/1
  CoG offset y/1 -> Car_Pose/8
  FaultInjectionLidar3/1 -> Fault Injection Listener Lidar 3/1
  [fi_camera_patch_b] -> Mux/7
  [fi_lidar_rain_reflectivity] -> Fault Injection Listener Lidar 2/7
  Demux2/4 -> Fault Injection Listener Camera 2/5
  Mux/1 -> Demux2/1, Demux1/1, Demux/1
  Fault Injection Listener Lidar 1/1 -> Fault Injection Lidar/5
  Demux/1 -> Fault Injection Listener Camera 1/2
  Demux1/7 -> Fault Injection Listener TL Camera/8
  Fault Injection Listener Camera 1/1 -> Fault Injection Camera1/4
  Fault Injection Listener Lidar 4/3 -> Fault Injection Lidar3/7
  Fault Injection Camera1/2 -> [camera1_g]
  CoG offset x/1 -> Car_Pose/7
  Demux1/4 -> Fault Injection Listener TL Camera/5
  [fi_lidar_rain_b] -> Fault Injection Listener Lidar 3/6
  Fault Injection Listener Lidar 3/8 -> Fault Injection Lidar2/12
  Demux/2 -> Fault Injection Listener Camera 1/3
  [fi_radar_phi_variance] -> Fault Injection Listener Radar/4
  [fi_lidar_rain_a] -> Fault Injection Listener Lidar 1/5
  [fi_camera_patch_size_x] -> Mux/3
  [fi_lidar_max_range] -> Fault Injection Listener Lidar 3/8
  Demux/3 -> Fault Injection Listener Camera 1/4
  [gt_camera2_r] -> Fault Injection Camera/1
  Demux/4 -> Fault Injection Listener Camera 1/5
  [fi_lidar_rain_reflectivity] -> Fault Injection Listener Lidar 1/7
  [fi_camera_patch_g] -> Mux/6
  [fi_lidar_rain_b] -> Fault Injection Listener Lidar 1/6
  Demux/6 -> Fault Injection Listener Camera 1/7
  Demux1/1 -> Fault Injection Listener TL Camera/2
  [gt_camera1_g] -> Fault Injection Camera1/2
  Demux1/6 -> Fault Injection Listener TL Camera/7
  Fault Injection Listener TL Camera/2 -> Fault Injection Camera2/5
  [fi_lidar_rain_b] -> Fault Injection Listener Lidar 4/6
  [Rotz] -> Car_Pose/6
  [fi_lidar_theta_variance] -> Fault Injection Listener Lidar 2/3
  Demux1/2 -> Fault Injection Listener TL Camera/3
  Demux2/7 -> Fault Injection Listener Camera 2/8
  [gt_camera2_b] -> Fault Injection Camera/3
  Fault Injection Listener TL Camera/8 -> Fault Injection Camera2/11
  [z] -> Car_Pose/3
  Fault Injection Listener Camera 2/6 -> Fault Injection Camera/9
  Fault Injection GNSS/1 -> [gnss_pose]
  Lidar Adapter2/1 -> [lidar3]
  Fault Injection Listener Camera 2/8 -> Fault Injection Camera/11
  [fi_lidar_range_variance] -> Fault Injection Listener Lidar 4/2
  [lidar4_range] -> Fault Injection Lidar3/1
  Fault Injection Listener TL Camera/1 -> Fault Injection Camera2/4
  Demux2/5 -> Fault Injection Listener Camera 2/6
  Demux2/3 -> Fault Injection Listener Camera 2/4
  [lidar2_intensity] -> Fault Injection Lidar1/4
  [fi_lidar_theta_variance] -> Fault Injection Listener Lidar 3/3
  Fault Injection Listener Lidar 4/8 -> Fault Injection Lidar3/12
  Demux1/5 -> Fault Injection Listener TL Camera/6
  [lidar3_phi] -> Fault Injection Lidar2/3
  Fault Injection Camera/1 -> [camera2_r]
  Demux2/6 -> Fault Injection Listener Camera 2/7
  Demux/5 -> Fault Injection Listener Camera 1/6
  [fi_lidar_range_variance] -> Fault Injection Listener Lidar 1/2
  [fi_lidar_max_range] -> Fault Injection Listener Lidar 2/8
  Demux2/1 -> Fault Injection Listener Camera 2/2
  [fi_radar_range_variance] -> Fault Injection Listener Radar/2
  [fi_lidar_rain_a] -> Fault Injection Listener Lidar 4/5
  [fi_lidar_rain_intensity] -> Fault Injection Listener Lidar 3/4
  [lidar4_intensity] -> Fault Injection Lidar3/4
  [fi_lidar_range_variance] -> Fault Injection Listener Lidar 2/2
  Lidar Adapter1/1 -> [lidar2]
  Fault Injection Listener Radar/1 -> Fault Injection Radar/5
  Fault Injection Radar/1 -> [radar_range]
  Fault Injection Listener Radar/2 -> Fault Injection Radar/6
  [fi_camera_patch_start_x] -> Mux/1
  Demux/7 -> Fault Injection Listener Camera 1/8
  Fault Injection Listener Camera 1/5 -> Fault Injection Camera1/8
  Demux2/2 -> Fault Injection Listener Camera 2/3
  [gt_radar] -> Bus Selector1/1
  [fi_lidar_max_range] -> Fault Injection Listener Lidar 4/8
  [fi_camera_patch_size_y] -> Mux/4
  Fault Injection Listener Camera 1/7 -> Fault Injection Camera1/10
  [fi_lidar_rain_reflectivity] -> Fault Injection Listener Lidar 4/7
  FaultInjectionLidar2/1 -> Fault Injection Listener Lidar 2/1
  [lidar1_intensity] -> Fault Injection Lidar/4
  Fault Injection Listener TL Camera/7 -> Fault Injection Camera2/10
  FaultInjectionLidar1/1 -> Fault Injection Listener Lidar 1/1
  Fault Injection Lidar/2 -> Lidar Adapter/3
  Bus Selector1/3 -> Fault Injection Radar/3  "<Phi[deg]>"
  Fault Injection Listener Lidar 2/2 -> Fault Injection Lidar1/6
  Fault Injection Lidar/1 -> Lidar Adapter/2
  Fault Injection Lidar/4 -> Lidar Adapter/5
  [base_link_pose] -> Fault Injection GNSS/1
  Car_Pose/1 -> [base_link_pose]
  Lidar Adapter/1 -> [lidar1]
  [Rotx] -> Car_Pose/4
  [fi_camera_patch_r] -> Mux/5
  [y] -> Car_Pose/2
  [fi_lidar_rain_intensity] -> Fault Injection Listener Lidar 2/4
  [fi_camera_patch_start_y] -> Mux/2
  [x] -> Car_Pose/1
  OrientationLidar3/1 -> Lidar Adapter2/1
  OrientationLidar1/1 -> Lidar Adapter/1
  Fault Injection Listener GNSS/1 -> Fault Injection GNSS/2
  Bus Selector1/1 -> Fault Injection Radar/1  "<Range[m]>"
  FaultInjectionGNSS/1 -> Fault Injection Listener GNSS/1
  Demux1/3 -> Fault Injection Listener TL Camera/4
  send_frequency_radar/1 -> frequency_evaluator_radar/1
  frequency_evaluator_camera2/1 -> [enable_camera2]
  send_frequency_tl_camera/1 -> frequency_evaluator_tl_camera/1
  frequency_evaluator_lidar/1 -> [enable_lidar]
  frequency_evaluator_gnss/1 -> [enable_gnss]
  frequency_evaluator_radar/1 -> [enable_radar]
  send_frequency_camera2/1 -> frequency_evaluator_camera2/1
  send_frequency_gnss/1 -> frequency_evaluator_gnss/1
  frequency_evaluator_tl_camera/1 -> [enable_tl_camera]
  send_frequency_camera1/1 -> frequency_evaluator_camera1/1
  frequency_evaluator_camera1/1 -> [enable_camera1]
  send_frequency_lidar/1 -> frequency_evaluator_lidar/1
  [enable_camera1] -> ROS Send Camera/Enable
  [enable_camera2] -> ROS Send Camera 2/Enable
  [enable_tl_camera] -> ROS Send Camera TL/Enable
  [enable_lidar] -> ROS Send Lidar/Enable
  [enable_radar] -> radarDetections/Enable
  [enable_gnss] -> ROS Send GNSS/Enable
  EnableSendGroundTruthPose/1 -> ROS Send Groud Truth Pose/Enable
  [base_link_pose] -> ROS Send Groud Truth Pose/1

== system adeye_lib/ROS Send Camera ==
  note: Because the image is RGB
  In1 : Inport
  In2 : Inport  Port=2
  In3 : Inport  Port=3
  Enable : EnablePort
  Assignment2 : Assignment  OutputInitialize=Specify size for each dimension in table  DiagnosticForDimensions=Warning  IndexOptions=Starting index (dialog)  Indices=1  OutputSizes=1000
  Blank Message3 : robotlib/Blank Message  messageClass=Message  entityType=sensor_msgs/Image  messageType=sensor_msgs/Image  SampleTime=inf
      settings: SourceProductBaseCode=RO
  Bus Assignment3 : BusAssignment  AssignedSignals=Height,Width,Encoding,Encoding_SL_Info.CurrentLength,Step,Data,Data_SL_Info.CurrentLength,Header.FrameId,Header.FrameId_SL_Info.CurrentLength
  Bus Selector2 : BusSelector  OutputSignals=Header.FrameId
  Constant19 : Constant  Value=uint8(['rgb8'])
  Constant20 : Constant  Value=uint8(['camera_1'])
  Constant25 : Constant  Value=3  OutDataTypeStr=Inherit: Inherit via back propagation
  Data Type Conversion1 : DataTypeConversion  OutDataTypeStr=uint8
  Math Function{,1..3} (4 alike) : Math  Operator=transpose  SaturateOnIntegerOverflow=on
  Matrix Concatenate : Concatenate  NumInputs=3  Mode=Multidimensional array  ConcatenateDimension=2
  Product : Product  OutDataTypeStr=uint32
  Publish1 : robotlib/Publish  topicSource=Specify your own  topic=/sensor/camera_1/image_raw  messageType=sensor_msgs/Image  messageQueueLength=1
      settings: SourceProductBaseCode=RO
  Reshape{1,17..19} (4 alike) : Reshape
  Variable Selector : dspindex/Variable Selector  NumInputs=1  rowsOrCols=Rows  IdxMode=Fixed  Elements=[1]  ZerOneIdxMode=One-based  errmode=Clip Index  FillMode=on  FillValues=0
  Variable Selector1 : dspindex/Variable Selector  NumInputs=1  rowsOrCols=Rows  IdxMode=Fixed  Elements=[1]  ZerOneIdxMode=One-based  errmode=Clip Index  FillMode=on  FillValues=0
  Width : Width
  Width1 : Width
  Width10 : Width  DataType=uint32
  Width5 : Width  DataType=uint32
  Width9 : Width  DataType=uint32
  wires:
  Reshape19/1 -> Matrix Concatenate/3
  Data Type Conversion1/1 -> Width9/1, Bus Assignment3/7
  Math Function/1 -> Variable Selector/1, Reshape17/1
  Constant25/1 -> Product/2
  Width/1 -> Bus Assignment3/2
  Width9/1 -> Bus Assignment3/8
  Bus Selector2/1 -> Assignment2/1  "<FrameId>"
  Product/1 -> Bus Assignment3/6
  Assignment2/1 -> Bus Assignment3/9
  Bus Assignment3/1 -> Publish1/1
  Constant19/1 -> Width5/1, Bus Assignment3/4
  Reshape18/1 -> Matrix Concatenate/2
  Width5/1 -> Bus Assignment3/5
  Reshape17/1 -> Matrix Concatenate/1
  Width10/1 -> Bus Assignment3/10
  Math Function2/1 -> Reshape19/1
  Constant20/1 -> Assignment2/2, Width10/1
  Width1/1 -> Bus Assignment3/3, Product/1
  Math Function1/1 -> Reshape18/1
  Blank Message3/1 -> Bus Selector2/1, Bus Assignment3/1
  In3/1 -> Math Function2/1
  In2/1 -> Math Function1/1
  In1/1 -> Variable Selector1/1, Math Function/1
  Reshape1/1 -> Data Type Conversion1/1
  Matrix Concatenate/1 -> Math Function3/1
  Math Function3/1 -> Reshape1/1
  Variable Selector/1 -> Width/1
  Variable Selector1/1 -> Width1/1

== system adeye_lib/ROS Send Camera 2 ==
  note: Because the image is RGB
  In1 : Inport
  In2 : Inport  Port=2
  In3 : Inport  Port=3
  Enable : EnablePort
  Assignment2 : Assignment  OutputInitialize=Specify size for each dimension in table  DiagnosticForDimensions=Warning  IndexOptions=Starting index (dialog)  Indices=1  OutputSizes=1000
  Blank Message3 : robotlib/Blank Message  messageClass=Message  entityType=sensor_msgs/Image  messageType=sensor_msgs/Image  SampleTime=inf
      settings: SourceProductBaseCode=RO
  Bus Assignment3 : BusAssignment  AssignedSignals=Height,Width,Encoding,Encoding_SL_Info.CurrentLength,Step,Data,Data_SL_Info.CurrentLength,Header.FrameId,Header.FrameId_SL_Info.CurrentLength
  Bus Selector2 : BusSelector  OutputSignals=Header.FrameId
  Constant19 : Constant  Value=uint8(['rgb8'])
  Constant20 : Constant  Value=uint8(['camera_2'])
  Constant25 : Constant  Value=3  OutDataTypeStr=Inherit: Inherit via back propagation
  Data Type Conversion1 : DataTypeConversion  OutDataTypeStr=uint8
  Math Function{,1..3} (4 alike) : Math  Operator=transpose  SaturateOnIntegerOverflow=on
  Matrix Concatenate : Concatenate  NumInputs=3  Mode=Multidimensional array  ConcatenateDimension=2
  Product : Product  OutDataTypeStr=uint32
  Publish1 : robotlib/Publish  topicSource=Specify your own  topic=/sensor/camera_2/image_raw  messageType=sensor_msgs/Image  messageQueueLength=1
      settings: SourceProductBaseCode=RO
  Reshape{1,17..19} (4 alike) : Reshape
  Variable Selector : dspindex/Variable Selector  NumInputs=1  rowsOrCols=Rows  IdxMode=Fixed  Elements=[1]  ZerOneIdxMode=One-based  errmode=Clip Index  FillMode=on  FillValues=0
  Variable Selector1 : dspindex/Variable Selector  NumInputs=1  rowsOrCols=Rows  IdxMode=Fixed  Elements=[1]  ZerOneIdxMode=One-based  errmode=Clip Index  FillMode=on  FillValues=0
  Width : Width
  Width1 : Width
  Width10 : Width  DataType=uint32
  Width5 : Width  DataType=uint32
  Width9 : Width  DataType=uint32
  wires:
  Reshape19/1 -> Matrix Concatenate/3
  Data Type Conversion1/1 -> Width9/1, Bus Assignment3/7
  Math Function/1 -> Variable Selector/1, Reshape17/1
  Constant25/1 -> Product/2
  Width/1 -> Bus Assignment3/2
  Width9/1 -> Bus Assignment3/8
  Bus Selector2/1 -> Assignment2/1  "<FrameId>"
  Product/1 -> Bus Assignment3/6
  Assignment2/1 -> Bus Assignment3/9
  Bus Assignment3/1 -> Publish1/1
  Constant19/1 -> Width5/1, Bus Assignment3/4
  Reshape18/1 -> Matrix Concatenate/2
  Width5/1 -> Bus Assignment3/5
  Reshape17/1 -> Matrix Concatenate/1
  Width10/1 -> Bus Assignment3/10
  Math Function2/1 -> Reshape19/1
  Constant20/1 -> Assignment2/2, Width10/1
  Width1/1 -> Bus Assignment3/3, Product/1
  Math Function1/1 -> Reshape18/1
  Blank Message3/1 -> Bus Selector2/1, Bus Assignment3/1
  In3/1 -> Math Function2/1
  In2/1 -> Math Function1/1
  In1/1 -> Variable Selector1/1, Math Function/1
  Reshape1/1 -> Data Type Conversion1/1
  Matrix Concatenate/1 -> Math Function3/1
  Math Function3/1 -> Reshape1/1
  Variable Selector/1 -> Width/1
  Variable Selector1/1 -> Width1/1
